simulink model "FOC_v2"  (R2017b)
settings: Solver=FixedStepDiscrete  StartTime=0.0  StopTime=10.0  FixedStep=0.0001  RelTol=1e-3
libraries: peTransforms x3
settings Model: Creator=EW  LastModifiedBy=EW
settings DataIOCC: LimitDataPoints=on  SaveFormat=Array
settings OptimizationCC: LifeSpan=1
settings DebuggingCC: SFUnexpectedBacktrackingDiag=warning  SFNoUnconditionalDefaultTransitionDiag=warning  SFExecutionAtInitializationDiag=none
settings HardwareCC: ProdBitPerPointer=32  ProdBitPerSizeT=32  ProdBitPerPtrDiffT=32  ProdLargestAtomicInteger=Long  ProdLargestAtomicFloat=Double  ProdIntDivRoundTo=Undefined  ProdWordSize=32  ProdHWDeviceType=ARM Compatible->ARM Cortex
settings ModelReferenceCC: PropagateSignalLabelsOutOfModel=off
settings SFSimCC: MATLABDynamicMemAlloc=off
settings RTWCC: SystemTargetFile=mbed.tlc  TemplateMakefile=mbed.tmf  Description=Mbed Target (Embedded Target)  TargetLang=C++
settings CodeAppCC: IgnoreCustomStorageClasses=off  StateflowObjectComments=on
settings STFCustomTargetCC: TargetLibSuffix=.a  GenerateSampleERTMain=on  CombineOutputUpdateFcns=on  ERTCustomFileBanners=on  SupportContinuousTime=off  SupportNonInlinedSFcns=off  RemoveResetFunc=on  MATLABClassNameForMDSCustomization=Simulink.SoftwareTarget.ERTCustomization  ModelStepFunctionPrototypeControlCompliant=on  GRTInterface=off  SystemTargetFile=mbed.tlc
settings ERTTargetCC: MultiwordLength=2048  GenerateSampleERTMain=on  ParMdlRefBuildCompliant=off  CompOptLevelCompliant=off  ConcurrentExecutionCompliant=off  CPPClassGenCompliant=off  UseToolchainInfoCompliant=off  ERTCustomFileTemplate=mbed_file_process.tlc  ConvertIfToSwitch=off  SuppressUnreachableDefaultCases=off
settings ConfigComp: CovMetricSettings=dw  CovHtmlReporting=on  CovSaveCumulativeToWorkspaceVar=on  CovSaveSingleToWorkspaceVar=on  CovExternalEMLEnable=off

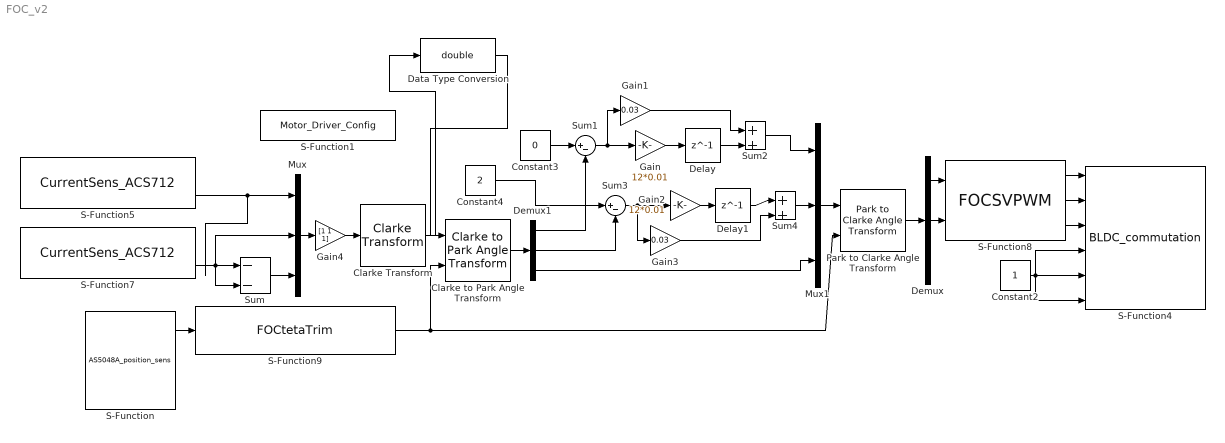
== system FOC_v2 ==
  Clarke Transform : peTransforms/Clarke Transform  PowerInvariant=on
  Clarke to Park Angle Transform : peTransforms/Clarke to Park Angle Transform  AxisAlignment=D-axis
  Constant2 : Constant  OutDataTypeStr=uint8
  Constant3 : Constant  Value=0
  Constant4 : Constant  Value=2
  Data Type Conversion : DataTypeConversion  OutDataTypeStr=double
  Delay : Delay  DelayLength=1  InitialCondition=0
  Delay1 : Delay  DelayLength=1  InitialCondition=0
  Demux : Demux  Outputs=3
  Demux1 : Demux  Outputs=3
  Gain : Gain  Gain=12*0.01
  Gain1 : Gain  Gain=0.03
  Gain2 : Gain  Gain=12*0.01
  Gain3 : Gain  Gain=0.03
  Gain4 : Gain  Gain=[1 1 1]
  Mux : Mux  Inputs=3
  Mux1 : Mux  Inputs=3
  Park to Clarke Angle Transform : peTransforms/Park to Clarke Angle Transform  AxisAlignment=D-axis
  S-Function : S-Function  Priority=0  FunctionName=AS5048A_position_sens  Parameters=SampleTime, uint8(PortName), uint8(PinNumber)  SFunctionDeploymentMode=off  EnableBusSupport=off  mask{PortName=C, PinNumber=8, SampleTime=-1}
      mask prompts: PinNumber "Pin Number:"; SampleTime "Sample time (-1 for inherited)"
      mask TypeOptions PortName: A | B | C | D | F | G | H | I | J | K
      mask TypeOptions PinNumber: 0 | 1 | 2 | 3 | 4 | 5 | 6 | 7 | 8 | 9 | 10 | 11 | 12 | 13 | 14 | 15
      mask Display:
      | disp('AS5048')
      | port_label('output',1,'RAW');
      | port_label('output',2,'rad');
      | port_label('output',3,'rad/s');
  S-Function1 : S-Function  Priority=1  FunctionName=Motor_Driver_Config  Parameters=uint8(PWMUport),uint8(PWMVport),uint8(PWMWport),uint8(PWMUpin),uint8(PWMVpin),uint8(PWMWpin),uint8(EnableUport),uint8(EnableVport),uint8(EnableWport),uint8(EnableUpin),uint8(EnableVpin),uint8(EnableWpin)  SFunctionDeploymentMode=off  EnableBusSupport=off  mask{PWMUport=A, PWMUpin=8, PWMVport=A, PWMVpin=9, PWMWport=A, PWMWpin=10, EnableUport=C, EnableUpin=10, EnableVport=C, EnableVpin=11, EnableWport=C, EnableWpin=12}
      mask prompts: PWMUport "PWM   U:      Port Name"; PWMUpin "Pin Number"; PWMVport "PWM   V:      Port Name"; PWMVpin "Pin Number"; PWMWport "PWM  W:      Port Name"; PWMWpin "Pin Number"; EnableUport "Enable  U:     Port Name"; EnableUpin "Pin Number"; EnableVport "Enable  V:     Port Name"; EnableVpin "Pin Number"; EnableWport "Enable W:     Port Name"; EnableWpin "Pin Number"
      mask TypeOptions PWMUport: A | B | C | D | E | F | G | H | I | J
      mask TypeOptions PWMUpin: 0 | 1 | 2 | 3 | 4 | 5 | 6 | 7 | 8 | 9 | 10 | 11 | 12 | 13 | 14 | 15
      mask TypeOptions PWMVport: A | B | C | D | E | F | G | H | I | J
      mask TypeOptions PWMVpin: 0 | 1 | 2 | 3 | 4 | 5 | 6 | 7 | 8 | 9 | 10 | 11 | 12 | 13 | 14 | 15
      mask TypeOptions PWMWport: A | B | C | D | E | F | G | H | I | J
      mask TypeOptions PWMWpin: 0 | 1 | 2 | 3 | 4 | 5 | 6 | 7 | 8 | 9 | 10 | 11 | 12 | 13 | 14 | 15
      mask TypeOptions EnableUport: A | B | C | D | E | F | G | H | I | J
      mask TypeOptions EnableUpin: 0 | 1 | 2 | 3 | 4 | 5 | 6 | 7 | 8 | 9 | 10 | 11 | 12 | 13 | 14 | 15
      mask TypeOptions EnableVport: A | B | C | D | E | F | G | H | I | J
      mask TypeOptions EnableVpin: 0 | 1 | 2 | 3 | 4 | 5 | 6 | 7 | 8 | 9 | 10 | 11 | 12 | 13 | 14 | 15
      mask TypeOptions EnableWport: A | B | C | D | E | F | G | H | I | J
      mask TypeOptions EnableWpin: 0 | 1 | 2 | 3 | 4 | 5 | 6 | 7 | 8 | 9 | 10 | 11 | 12 | 13 | 14 | 15
  S-Function4 : S-Function  FunctionName=BLDC_commutation  Parameters=SampleTime  SFunctionDeploymentMode=off  EnableBusSupport=off  mask{SampleTime=-1}
      mask prompts: SampleTime "Sample time (-1 for inherited):"
      mask Display:
      | disp(['BLDC Commutation'])
      | 
      | port_label('input',1,'PWM U');
      | port_label('input',2,'PWM V');
      | port_label('input',3,'PWM W');
      | port_label('input',4,'Enable U');
      | port_label('input',5,'Enable V');
      | port_label('input',6,'Enable W');
  S-Function5 : S-Function  FunctionName=CurrentSens_ACS712  Parameters=SampleTime,uint8(PortName),uint8(PinNumber), single(Vref),single(Sensitivity)  SFunctionDeploymentMode=off  EnableBusSupport=off  mask{PortName=C, PinNumber=4, Vref=3.3, Sensitivity=0.185, SampleTime=-1}
      mask prompts: PortName "Port Name:"; PinNumber "Pin Number"; Vref "Vref [V]"; Sensitivity "Sensitivity [V per A]"; SampleTime "Sample time (-1 for inherited)"
      mask TypeOptions PortName: A | B | C | D | E | F | G | H | I | J | K
      mask TypeOptions PinNumber: 0 | 1 | 2 | 3 | 4 | 5 | 6 | 7 | 8 | 9 | 10 | 11 | 12 | 13 | 14 | 15
      mask Display:
      | disp('Current Sens ACS712ELC')
      | port_label('output',1,'RAW');
      | port_label('output',2,'Current');
  S-Function7 : S-Function  FunctionName=CurrentSens_ACS712  Parameters=SampleTime,uint8(PortName),uint8(PinNumber), single(Vref),single(Sensitivity)  SFunctionDeploymentMode=off  EnableBusSupport=off  mask{PortName=C, PinNumber=5, Vref=3.3, Sensitivity=0.185, SampleTime=-1}
      mask prompts: PortName "Port Name:"; PinNumber "Pin Number"; Vref "Vref [V]"; Sensitivity "Sensitivity [V per A]"; SampleTime "Sample time (-1 for inherited)"
      mask TypeOptions PortName: A | B | C | D | E | F | G | H | I | J | K
      mask TypeOptions PinNumber: 0 | 1 | 2 | 3 | 4 | 5 | 6 | 7 | 8 | 9 | 10 | 11 | 12 | 13 | 14 | 15
      mask Display:
      | disp('Current Sens ACS712ELC')
      | port_label('output',1,'RAW');
      | port_label('output',2,'Current');
  S-Function8 : S-Function  FunctionName=FOCSVPWM  Parameters=SampleTime  SFunctionDeploymentMode=off  EnableBusSupport=off  mask{SampleTime=-1}
      mask prompts: SampleTime "Sample time(-1 for inherited):"
      mask Display:
      | disp('FOC\nSVPWM')
      | port_label('output',1,'duty U');
      | port_label('output',2,'duty V');
      | port_label('output',3,'duty W');
      | port_label('input',1,'alpha');
      | port_label('input',2,'beta');
  S-Function9 : S-Function  FunctionName=FOCtetaTrim  Parameters=SampleTime,uint16(trim)  SFunctionDeploymentMode=off  EnableBusSupport=off  mask{trim=36, SampleTime=-1}
      mask prompts: SampleTime "Sample time(-1 for inherited):"
      mask help: Trim the angle to be 0 on phase U and establish a virtual angle for a 22 pole machine for FOC
      mask Display:
      | disp('Angle-Trim\nphysical2electric\n22 pole Machine');
      | port_label('output',1,'teta[rad]');
      | port_label('input',1,'teta[raw]');
  Sum : Sum  Inputs=|--
  Sum1 : Sum  Inputs=|+-
  Sum2 : Sum  Inputs=|++
  Sum3 : Sum  Inputs=|+-
  Sum4 : Sum  Inputs=|++
  wires:
  S-Function7/2 -> Mux/2, Sum/2
  Constant2/1 -> S-Function4/6, S-Function4/5, S-Function4/4
  S-Function9/1 -> Park to Clarke Angle Transform/2, Clarke to Park Angle Transform/2
  Demux1/1 -> Sum1/2
  Constant3/1 -> Sum1/1
  Sum1/1 -> Gain1/1, Gain/1
  Gain/1 -> Delay/1
  Demux1/3 -> Mux1/3
  Delay/1 -> Sum2/2
  Gain1/1 -> Sum2/1
  Sum2/1 -> Mux1/1
  Gain2/1 -> Delay1/1
  Sum3/1 -> Gain2/1, Gain3/1
  Constant4/1 -> Sum3/1
  Delay1/1 -> Sum4/1
  Gain3/1 -> Sum4/2
  Sum4/1 -> Mux1/2
  Demux1/2 -> Sum3/2
  Mux1/1 -> Park to Clarke Angle Transform/1
  Demux/1 -> S-Function8/1
  Demux/2 -> S-Function8/2
  S-Function/1 -> S-Function9/1
  S-Function8/1 -> S-Function4/1
  S-Function8/2 -> S-Function4/2
  S-Function8/3 -> S-Function4/3
  Sum/1 -> Mux/3
  S-Function5/2 -> Mux/1, Sum/1
  Gain4/1 -> Clarke Transform/1
  Mux/1 -> Gain4/1
  Clarke to Park Angle Transform/1 -> Demux1/1
  Park to Clarke Angle Transform/1 -> Demux/1
  Clarke Transform/1 -> Data Type Conversion/1
  Data Type Conversion/1 -> Clarke to Park Angle Transform/1
